simulink model "pidCascade_struc2_Analysis_PCTOP"  (R2017b)
settings: Solver=ode45  StartTime=0.0  StopTime=10.0  RelTol=1e-3
values from neighbouring files (symbols this model uses):
  A = [-0.00336681378328 0.00605987984547 -0.0270035472853 0 0 0 -0.00326756764621 0.0184340188312 0.000574501584014 0.00856952845414 0.00856180728817 -0.0456898724713 ... (100 elements, 10x10)]    [jacobians.mat]    (also in jacobians_SelfOpt_z5.mat = [-0.0025 0.00333333333333 0 0 0 0 0 0 0 0 0 0 ... (196 eleme; jacobians_struc2.mat = [-0.00291491994724 0.00530962585305 -0.0226365156276 0 0 0 -; jacobians_struc2_Opt.mat = [-0.00166666666667 2066.16160269 2.24994189684 -2.5145068292; jacobians_struc2_z5 (Esmaeil Jahanshahi's conflicted copy 2017-05-14).mat = [0 0 11336267.4269 38.4435006212 -45.2522810388 198.40758894)
  B = [2.78217322635 -3.13684380945 10.470572963 0 0 0 1.64365732825 -9.27271090354 -0.288986745157 -4.31065849843 0 0 ... (50 elements, 10x5)]    [jacobians.mat]    (also in jacobians_SelfOpt_z5.mat = [0 0 0 -1.41162624529e-07 3.97826884955e-06 0 0 0 0 0 1.7156; jacobians_struc2.mat = [2.4235380092 -2.52676653138 7.52074497057 0 0 0 1.314279160; jacobians_struc2_Opt.mat = [0.00166666666667 0 0 0 0 0 0 0 0 0 0 0 ... (75 elements, 15; jacobians_struc2_z5 (Esmaeil Jahanshahi's conflicted copy 2017-05-14).mat = [0 0.0025 0 0 0 0 0 0 0 0 0 0 ... (85 elements, 17x5)])
  C = [1987.64160023 0 0 0 0 0 10193.8151816 0 0 0 0 224.929909527 ... (50 elements, 5x10)]    [jacobians.mat]    (also in jacobians_SelfOpt_z5.mat = [0 0 0 0 0 0 0 0 0 0 0 0 ... (182 elements, 13x14)]; jacobians_struc2.mat = [1987.64160023 0 0 0 0 0 0 9760.79528905 0 0 0 0 ... (60 ele; jacobians_struc2_Opt.mat = [0 0 0 0 0 0 0 0 0 0 0 0 ... (90 elements, 6x15)]; jacobians_struc2_z5 (Esmaeil Jahanshahi's conflicted copy 2017-05-14).mat = [0 0 0 0 0 0 0 0 0 0 0 0 ... (102 elements, 6x17)])
  D = [0 0 0 0 0 0 0 0 0 0 0 0 ... (25 elements, 5x5)]    [jacobians.mat]    (also in jacobians_SelfOpt_z5.mat = [0 0 0 0 0 0 0 0 -1.52061884955e-06 0 -1.36710622502e-06 0 .; jacobians_struc2.mat = [0 0 0 0 0 0 0 0 0 0 0 0 ... (30 elements, 6x5)]; jacobians_struc2_Opt.mat = [0 0 0 0 0 0 0 0 0 0 0 0 ... (30 elements, 6x5)]; jacobians_struc2_z5 (Esmaeil Jahanshahi's conflicted copy 2017-05-14).mat = [0 0 0 0 0 0 0 0 0 0 0 0 ... (30 elements, 6x5)])
  PCA1Kc = -3e-05    [TuningValues.mat]    (also in pidCascadeTestStability.m = -1e-05; pidCascade_struc2_TestStability_PCA1.m)
  PCA1Tf = 0    [TuningValues.mat]    (also in pidCascadeTestStability.m = 1; pidCascade_struc2_TestStability_PCA1.m)
  PCA1Ti = 600    [TuningValues.mat]    (also in pidCascadeTestStability.m; pidCascade_struc2_TestStability_PCA1.m)
  PCA2Kc = -3e-05    [TuningValues.mat]    (also in pidCascadeTestStability.m = -1e-05; pidCascade_struc2_TestStability_PCA2.m)
  PCA2Tf = 0    [TuningValues.mat]    (also in pidCascadeTestStability.m = 1; pidCascade_struc2_TestStability_PCA2.m)
  PCA2Ti = 600    [TuningValues.mat]    (also in pidCascadeTestStability.m; pidCascade_struc2_TestStability_PCA2.m)
  PCINLKc = -2e-06    [TuningValues.mat]    (also in pidCascadeTestStability.m; pidCascade_struc2_TestStability_PCINL.m)
  PCINLTf = 0    [TuningValues.mat]    (also in pidCascadeTestStability.m = 1; pidCascade_struc2_TestStability_PCINL.m)
  PCINLTi = 300    [TuningValues.mat]    (also in pidCascadeTestStability.m = 900; pidCascade_struc2_TestStability_PCINL.m)
  PCT1Kc = 4e-09    [TuningValues.mat]    (also in pidCascadeTestStability.m = 4e-08; pidCascade_struc2_TestStability_PCT1.m)
  PCT1Tf = 0    [TuningValues.mat]    (also in pidCascadeTestStability.m = 900; pidCascade_struc2_TestStability_PCT1.m)
  PCT1Ti = 100    [TuningValues.mat]    (also in pidCascadeTestStability.m = 900; pidCascade_struc2_TestStability_PCT1.m)
  PCT2Kc = 4e-09    [TuningValues.mat]    (also in pidCascadeTestStability.m = 4e-08; pidCascade_struc2_TestStability_PCT2.m)
  PCT2Tf = 0    [TuningValues.mat]    (also in pidCascadeTestStability.m = 900; pidCascade_struc2_TestStability_PCT2.m)
  PCT2Ti = 100    [TuningValues.mat]    (also in pidCascadeTestStability.m = 900; pidCascade_struc2_TestStability_PCT2.m)
libraries: simulink x5
settings Model: Creator=Administrator  LastModifiedBy=Administrator
settings DataIOCC: LimitDataPoints=on  SaveFormat=Array  SignalLoggingSaveFormat=ModelDataLogs
settings OptimizationCC: BlockReduction=off  BooleanDataType=off  LifeSpan=inf
settings DebuggingCC: SaveWithParameterizedLinksMsg=none  UnderspecifiedInitializationDetection=Classic  MergeDetectMultiDrivingBlocksExec=none  SignalResolutionControl=TryResolveAllWithWarning  MultiTaskDSMMsg=warning  MultiTaskCondExecSysMsg=none  AllowSymbolicDim=off  StateNameClashWarn=warning  SFUnexpectedBacktrackingDiag=warning  SFNoUnconditionalDefaultTransitionDiag=warning  SFExecutionAtInitializationDiag=none
settings HardwareCC: ProdBitPerPointer=32  ProdBitPerSizeT=32  ProdBitPerPtrDiffT=32  ProdLargestAtomicFloat=None  ProdIntDivRoundTo=Undefined  ProdEndianess=Unspecified  ProdWordSize=32  ProdHWDeviceType=32-bit Generic  TargetUnknown=on
settings ModelReferenceCC: PropagateSignalLabelsOutOfModel=off
settings CodeAppCC: StateflowObjectComments=on
settings GRTTargetCC: TargetLangStandard=C89/C90 (ANSI)  GeneratePreprocessorConditionals=Disable all
settings ConfigComp: CovMetricSettings=dw  CovHtmlReporting=on  CovSaveCumulativeToWorkspaceVar=on  CovSaveSingleToWorkspaceVar=on  CovExternalEMLEnable=off

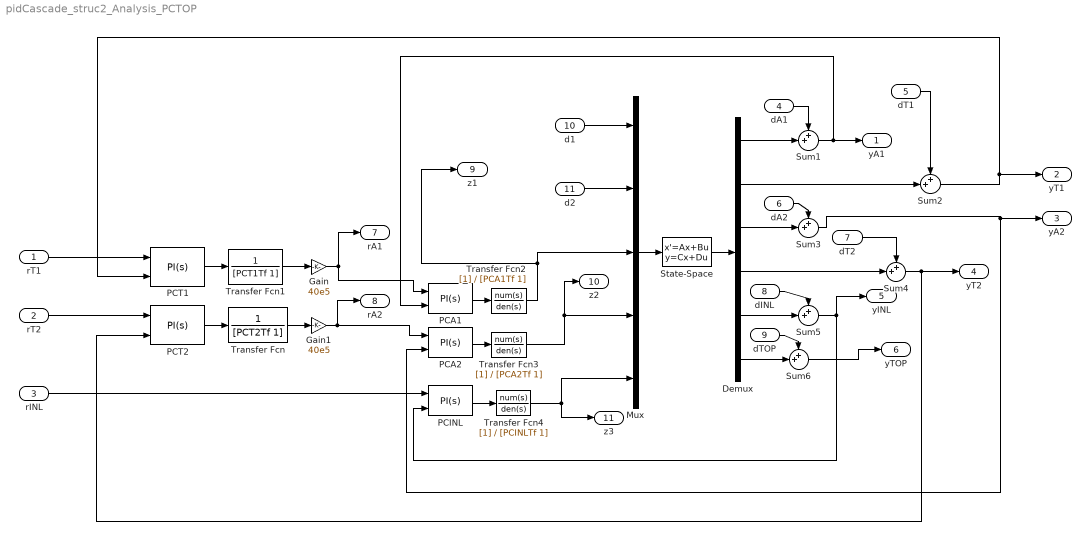
== system pidCascade_struc2_Analysis_PCTOP ==
  rT1 : Inport
  rT2 : Inport  Port=2
  rINL : Inport  Port=3
  dA1 : Inport  Port=4
  dT1 : Inport  Port=5
  dA2 : Inport  Port=6
  dT2 : Inport  Port=7
  dINL : Inport  Port=8
  dTOP : Inport  Port=9
  d1 : Inport  Port=10
  d2 : Inport  Port=11
  Demux : Demux  Outputs=6
  Gain : Gain  Gain=40e5
  Gain1 : Gain  Gain=40e5
  Mux : Mux  Inputs=5
  PCA1 : simulink/Continuous/PID Controller (2DOF)  Controller=PI  TimeDomain=Continuous-time  SampleTime=-1  IntegratorMethod=Forward Euler  FilterMethod=Forward Euler  Form=Ideal  UseFilter=on  ControllerParametersSource=internal  P=PCA1Kc  I=1/PCA1Ti  D=0  N=100  b=1  c=1  InitialConditionSource=internal  InitialConditionForIntegrator=0  InitialConditionForFilter=0  ExternalReset=none  LimitOutput=off  UpperSaturationLimit=inf  LowerSaturationLimit=-inf  LinearizeAsGain=on  AntiWindupMode=none  Kb=1  TrackingMode=off  Kt=1  PParamMin=[]  PParamMax=[]  IParamMin=[]  IParamMax=[]  DParamMin=[]  DParamMax=[]  NParamMin=[]  NParamMax=[]  bParamMin=[]  bParamMax=[]  cParamMin=[]  cParamMax=[]  KbParamMin=[]  KbParamMax=[]  KtParamMin=[]  KtParamMax=[]  POutMin=[]  POutMax=[]  IOutMin=[]  IOutMax=[]  DOutMin=[]  DOutMax=[]  NOutMin=[]  NOutMax=[]  bOutMin=[]  bOutMax=[]  cOutMin=[]  cOutMax=[]  KbOutMin=[]  KbOutMax=[]  KtOutMin=[]  KtOutMax=[]  IntegratorOutMin=[]  IntegratorOutMax=[]  FilterOutMin=[]  FilterOutMax=[]  SumOutMin=[]  SumOutMax=[]  Sum1OutMin=[]  Sum1OutMax=[]  Sum2OutMin=[]  Sum2OutMax=[]  Sum3OutMin=[]  Sum3OutMax=[]  SumI1OutMin=[]  SumI1OutMax=[]  SumI2OutMin=[]  SumI2OutMax=[]  SumI3OutMin=[]  SumI3OutMax=[]  SumDOutMin=[]  SumDOutMax=[]  SaturationOutMin=[]  SaturationOutMax=[]  IntegratorContinuousStateAttributes=''  IntegratorStateMustResolveToSignalObject=off  IntegratorRTWStateStorageClass=Auto  FilterContinuousStateAttributes=''  FilterStateMustResolveToSignalObject=off  FilterRTWStateStorageClass=Auto  DifferentiatorICPrevScaledInput=0  DifferentiatorOutMin=[]  DifferentiatorOutMax=[]  InitialConditionSetting=State (most efficient)  FilterDiffOutCoefMin=[]  FilterDiffOutCoefMax=[]  SumDenOutMin=[]  SumDenOutMax=[]  SumNumOutMin=[]  SumNumOutMax=[]  ReciprocalOutMin=[]  ReciprocalOutMax=[]  DivideOutMin=[]  DivideOutMax=[]  TunerSelectOption=Transfer Function Based (PID Tuner App)
  PCA2 : simulink/Continuous/PID Controller (2DOF)  Controller=PI  TimeDomain=Continuous-time  SampleTime=-1  IntegratorMethod=Forward Euler  FilterMethod=Forward Euler  Form=Ideal  UseFilter=on  ControllerParametersSource=internal  P=PCA2Kc  I=1/PCA2Ti  D=0  N=100  b=1  c=1  InitialConditionSource=internal  InitialConditionForIntegrator=0  InitialConditionForFilter=0  ExternalReset=none  LimitOutput=off  UpperSaturationLimit=inf  LowerSaturationLimit=-inf  LinearizeAsGain=on  AntiWindupMode=none  Kb=1  TrackingMode=off  Kt=1  PParamMin=[]  PParamMax=[]  IParamMin=[]  IParamMax=[]  DParamMin=[]  DParamMax=[]  NParamMin=[]  NParamMax=[]  bParamMin=[]  bParamMax=[]  cParamMin=[]  cParamMax=[]  KbParamMin=[]  KbParamMax=[]  KtParamMin=[]  KtParamMax=[]  POutMin=[]  POutMax=[]  IOutMin=[]  IOutMax=[]  DOutMin=[]  DOutMax=[]  NOutMin=[]  NOutMax=[]  bOutMin=[]  bOutMax=[]  cOutMin=[]  cOutMax=[]  KbOutMin=[]  KbOutMax=[]  KtOutMin=[]  KtOutMax=[]  IntegratorOutMin=[]  IntegratorOutMax=[]  FilterOutMin=[]  FilterOutMax=[]  SumOutMin=[]  SumOutMax=[]  Sum1OutMin=[]  Sum1OutMax=[]  Sum2OutMin=[]  Sum2OutMax=[]  Sum3OutMin=[]  Sum3OutMax=[]  SumI1OutMin=[]  SumI1OutMax=[]  SumI2OutMin=[]  SumI2OutMax=[]  SumI3OutMin=[]  SumI3OutMax=[]  SumDOutMin=[]  SumDOutMax=[]  SaturationOutMin=[]  SaturationOutMax=[]  IntegratorContinuousStateAttributes=''  IntegratorStateMustResolveToSignalObject=off  IntegratorRTWStateStorageClass=Auto  FilterContinuousStateAttributes=''  FilterStateMustResolveToSignalObject=off  FilterRTWStateStorageClass=Auto  DifferentiatorICPrevScaledInput=0  DifferentiatorOutMin=[]  DifferentiatorOutMax=[]  InitialConditionSetting=State (most efficient)  FilterDiffOutCoefMin=[]  FilterDiffOutCoefMax=[]  SumDenOutMin=[]  SumDenOutMax=[]  SumNumOutMin=[]  SumNumOutMax=[]  ReciprocalOutMin=[]  ReciprocalOutMax=[]  DivideOutMin=[]  DivideOutMax=[]  TunerSelectOption=Transfer Function Based (PID Tuner App)
  PCINL : simulink/Continuous/PID Controller (2DOF)  Controller=PI  TimeDomain=Continuous-time  SampleTime=-1  IntegratorMethod=Forward Euler  FilterMethod=Forward Euler  Form=Ideal  UseFilter=on  ControllerParametersSource=internal  P=PCINLKc  I=1/PCINLTi  D=0  N=100  b=1  c=1  InitialConditionSource=internal  InitialConditionForIntegrator=0  InitialConditionForFilter=0  ExternalReset=none  LimitOutput=off  UpperSaturationLimit=inf  LowerSaturationLimit=-inf  LinearizeAsGain=on  AntiWindupMode=none  Kb=1  TrackingMode=off  Kt=1  PParamMin=[]  PParamMax=[]  IParamMin=[]  IParamMax=[]  DParamMin=[]  DParamMax=[]  NParamMin=[]  NParamMax=[]  bParamMin=[]  bParamMax=[]  cParamMin=[]  cParamMax=[]  KbParamMin=[]  KbParamMax=[]  KtParamMin=[]  KtParamMax=[]  POutMin=[]  POutMax=[]  IOutMin=[]  IOutMax=[]  DOutMin=[]  DOutMax=[]  NOutMin=[]  NOutMax=[]  bOutMin=[]  bOutMax=[]  cOutMin=[]  cOutMax=[]  KbOutMin=[]  KbOutMax=[]  KtOutMin=[]  KtOutMax=[]  IntegratorOutMin=[]  IntegratorOutMax=[]  FilterOutMin=[]  FilterOutMax=[]  SumOutMin=[]  SumOutMax=[]  Sum1OutMin=[]  Sum1OutMax=[]  Sum2OutMin=[]  Sum2OutMax=[]  Sum3OutMin=[]  Sum3OutMax=[]  SumI1OutMin=[]  SumI1OutMax=[]  SumI2OutMin=[]  SumI2OutMax=[]  SumI3OutMin=[]  SumI3OutMax=[]  SumDOutMin=[]  SumDOutMax=[]  SaturationOutMin=[]  SaturationOutMax=[]  IntegratorContinuousStateAttributes=''  IntegratorStateMustResolveToSignalObject=off  IntegratorRTWStateStorageClass=Auto  FilterContinuousStateAttributes=''  FilterStateMustResolveToSignalObject=off  FilterRTWStateStorageClass=Auto  DifferentiatorICPrevScaledInput=0  DifferentiatorOutMin=[]  DifferentiatorOutMax=[]  InitialConditionSetting=State (most efficient)  FilterDiffOutCoefMin=[]  FilterDiffOutCoefMax=[]  SumDenOutMin=[]  SumDenOutMax=[]  SumNumOutMin=[]  SumNumOutMax=[]  ReciprocalOutMin=[]  ReciprocalOutMax=[]  DivideOutMin=[]  DivideOutMax=[]  TunerSelectOption=Transfer Function Based (PID Tuner App)
  PCT1 : simulink/Continuous/PID Controller (2DOF)  Controller=PI  TimeDomain=Continuous-time  SampleTime=-1  IntegratorMethod=Forward Euler  FilterMethod=Forward Euler  Form=Ideal  UseFilter=on  ControllerParametersSource=internal  P=PCT1Kc  I=1/PCT1Ti  D=0  N=100  b=1  c=1  InitialConditionSource=internal  InitialConditionForIntegrator=0  InitialConditionForFilter=0  ExternalReset=none  LimitOutput=off  UpperSaturationLimit=inf  LowerSaturationLimit=-inf  LinearizeAsGain=on  AntiWindupMode=none  Kb=1  TrackingMode=off  Kt=1  PParamMin=[]  PParamMax=[]  IParamMin=[]  IParamMax=[]  DParamMin=[]  DParamMax=[]  NParamMin=[]  NParamMax=[]  bParamMin=[]  bParamMax=[]  cParamMin=[]  cParamMax=[]  KbParamMin=[]  KbParamMax=[]  KtParamMin=[]  KtParamMax=[]  POutMin=[]  POutMax=[]  IOutMin=[]  IOutMax=[]  DOutMin=[]  DOutMax=[]  NOutMin=[]  NOutMax=[]  bOutMin=[]  bOutMax=[]  cOutMin=[]  cOutMax=[]  KbOutMin=[]  KbOutMax=[]  KtOutMin=[]  KtOutMax=[]  IntegratorOutMin=[]  IntegratorOutMax=[]  FilterOutMin=[]  FilterOutMax=[]  SumOutMin=[]  SumOutMax=[]  Sum1OutMin=[]  Sum1OutMax=[]  Sum2OutMin=[]  Sum2OutMax=[]  Sum3OutMin=[]  Sum3OutMax=[]  SumI1OutMin=[]  SumI1OutMax=[]  SumI2OutMin=[]  SumI2OutMax=[]  SumI3OutMin=[]  SumI3OutMax=[]  SumDOutMin=[]  SumDOutMax=[]  SaturationOutMin=[]  SaturationOutMax=[]  IntegratorContinuousStateAttributes=''  IntegratorStateMustResolveToSignalObject=off  IntegratorRTWStateStorageClass=Auto  FilterContinuousStateAttributes=''  FilterStateMustResolveToSignalObject=off  FilterRTWStateStorageClass=Auto  DifferentiatorICPrevScaledInput=0  DifferentiatorOutMin=[]  DifferentiatorOutMax=[]  InitialConditionSetting=State (most efficient)  FilterDiffOutCoefMin=[]  FilterDiffOutCoefMax=[]  SumDenOutMin=[]  SumDenOutMax=[]  SumNumOutMin=[]  SumNumOutMax=[]  ReciprocalOutMin=[]  ReciprocalOutMax=[]  DivideOutMin=[]  DivideOutMax=[]  TunerSelectOption=Transfer Function Based (PID Tuner App)
  PCT2 : simulink/Continuous/PID Controller (2DOF)  Controller=PI  TimeDomain=Continuous-time  SampleTime=-1  IntegratorMethod=Forward Euler  FilterMethod=Forward Euler  Form=Ideal  UseFilter=on  ControllerParametersSource=internal  P=PCT2Kc  I=1/PCT2Ti  D=0  N=100  b=1  c=1  InitialConditionSource=internal  InitialConditionForIntegrator=0  InitialConditionForFilter=0  ExternalReset=none  LimitOutput=off  UpperSaturationLimit=inf  LowerSaturationLimit=-inf  LinearizeAsGain=on  AntiWindupMode=none  Kb=1  TrackingMode=off  Kt=1  PParamMin=[]  PParamMax=[]  IParamMin=[]  IParamMax=[]  DParamMin=[]  DParamMax=[]  NParamMin=[]  NParamMax=[]  bParamMin=[]  bParamMax=[]  cParamMin=[]  cParamMax=[]  KbParamMin=[]  KbParamMax=[]  KtParamMin=[]  KtParamMax=[]  POutMin=[]  POutMax=[]  IOutMin=[]  IOutMax=[]  DOutMin=[]  DOutMax=[]  NOutMin=[]  NOutMax=[]  bOutMin=[]  bOutMax=[]  cOutMin=[]  cOutMax=[]  KbOutMin=[]  KbOutMax=[]  KtOutMin=[]  KtOutMax=[]  IntegratorOutMin=[]  IntegratorOutMax=[]  FilterOutMin=[]  FilterOutMax=[]  SumOutMin=[]  SumOutMax=[]  Sum1OutMin=[]  Sum1OutMax=[]  Sum2OutMin=[]  Sum2OutMax=[]  Sum3OutMin=[]  Sum3OutMax=[]  SumI1OutMin=[]  SumI1OutMax=[]  SumI2OutMin=[]  SumI2OutMax=[]  SumI3OutMin=[]  SumI3OutMax=[]  SumDOutMin=[]  SumDOutMax=[]  SaturationOutMin=[]  SaturationOutMax=[]  IntegratorContinuousStateAttributes=''  IntegratorStateMustResolveToSignalObject=off  IntegratorRTWStateStorageClass=Auto  FilterContinuousStateAttributes=''  FilterStateMustResolveToSignalObject=off  FilterRTWStateStorageClass=Auto  DifferentiatorICPrevScaledInput=0  DifferentiatorOutMin=[]  DifferentiatorOutMax=[]  InitialConditionSetting=State (most efficient)  FilterDiffOutCoefMin=[]  FilterDiffOutCoefMax=[]  SumDenOutMin=[]  SumDenOutMax=[]  SumNumOutMin=[]  SumNumOutMax=[]  ReciprocalOutMin=[]  ReciprocalOutMax=[]  DivideOutMin=[]  DivideOutMax=[]  TunerSelectOption=Transfer Function Based (PID Tuner App)
  State-Space : StateSpace  A=A  B=B  C=C  D=D  InitialCondition=0
  Sum{1..6} (6 alike) : Sum  Inputs=++|
  Transfer Fcn : TransferFcn  Denominator=[PCT2Tf 1]
  Transfer Fcn1 : TransferFcn  Denominator=[PCT1Tf 1]
  Transfer Fcn2 : TransferFcn  Denominator=[PCA1Tf 1]
  Transfer Fcn3 : TransferFcn  Denominator=[PCA2Tf 1]
  Transfer Fcn4 : TransferFcn  Denominator=[PCINLTf 1]
  yA1 : Outport
  yT1 : Outport  Port=2
  yA2 : Outport  Port=3
  yT2 : Outport  Port=4
  yINL : Outport  Port=5
  yTOP : Outport  Port=6
  rA1 : Outport  Port=7
  rA2 : Outport  Port=8
  z1 : Outport  Port=9
  z2 : Outport  Port=10
  z3 : Outport  Port=11
  wires:
  State-Space/1 -> Demux/1
  Mux/1 -> State-Space/1
  Demux/1 -> Sum1/2
  Demux/2 -> Sum2/2
  Demux/3 -> Sum3/2
  PCA1/1 -> Transfer Fcn2/1
  PCA2/1 -> Transfer Fcn3/1
  Transfer Fcn1/1 -> Gain/1
  Transfer Fcn/1 -> Gain1/1
  Gain/1 -> rA1/1, PCA1/1
  PCT1/1 -> Transfer Fcn1/1
  Gain1/1 -> rA2/1, PCA2/1
  PCT2/1 -> Transfer Fcn/1
  rT1/1 -> PCT1/1
  rT2/1 -> PCT2/1
  Transfer Fcn2/1 -> Mux/3, z1/1
  Transfer Fcn3/1 -> z2/1, Mux/4
  PCINL/1 -> Transfer Fcn4/1
  dA1/1 -> Sum1/1
  Sum1/1 -> yA1/1, PCA1/2
  Sum2/1 -> yT1/1, PCT1/2
  dT1/1 -> Sum2/1
  dA2/1 -> Sum3/1
  Sum3/1 -> yA2/1, PCA2/2
  Demux/4 -> Sum4/2
  Sum4/1 -> yT2/1, PCT2/2
  dT2/1 -> Sum4/1
  Demux/5 -> Sum5/2
  Sum5/1 -> yINL/1, PCINL/2
  dINL/1 -> Sum5/1
  Sum6/1 -> yTOP/1
  rINL/1 -> PCINL/1
  Demux/6 -> Sum6/2
  dTOP/1 -> Sum6/1
  Transfer Fcn4/1 -> Mux/5, z3/1
  d2/1 -> Mux/2
  d1/1 -> Mux/1
